simulink model "DPGandLQRIdentHandK"  (R2025b)
settings: Solver=VariableStepAuto  StartTime=0.0  StopTime=60000  FixedStep=1e-3  MaxStep=1e-3  RelTol=1e-3
values from neighbouring files (symbols this model uses):
  A = [1.0000    0.0099 ... (first row only)    [DPGandLQRIdentHandK.m]    (also in DPGandLQR_usingDlfevel.m = [1.0000, 0.0099; DPGandLQRsimOnlyIdentH.m)
  B = [4.9503e-05 ... (first row only)    [DPGandLQRIdentHandK.m]    (also in DPGandLQR_usingDlfevel.m; DPGandLQRsimOnlyIdentH.m)
  C = eye(size(A))    [DPGandLQRIdentHandK.m]    (also in DPGandLQRsimOnlyIdentH.m)
  H_critic = (H_critic + H_critic') / 2    [DPGandLQRIdentHandK.m]    (also in DPGandLQR_usingDlfevel.m = 0.5 * (H_critic + H_critic'); DPGandLQRsimOnlyIdentH.m)
  Herror = [1 1 1;1  1 1;1 1 1]*20    [DPGandLQRIdentHandK.m]    (also in DPGandLQRsimOnlyIdentH.m)
  Q = eye(2)    [DPGandLQRIdentHandK.m]    (also in DPGandLQR_usingDlfevel.m; DPGandLQRsimOnlyIdentH.m)
  R = 1    [DPGandLQRIdentHandK.m]    (also in DPGandLQR_usingDlfevel.m; DPGandLQRsimOnlyIdentH.m)
undefined symbols (not defined in the file or in its folder): K_lqr, magnitude, P_star
libraries: simulink x2
settings Model: PacingRate=1000  Creator=17547  LastModifiedBy=17547

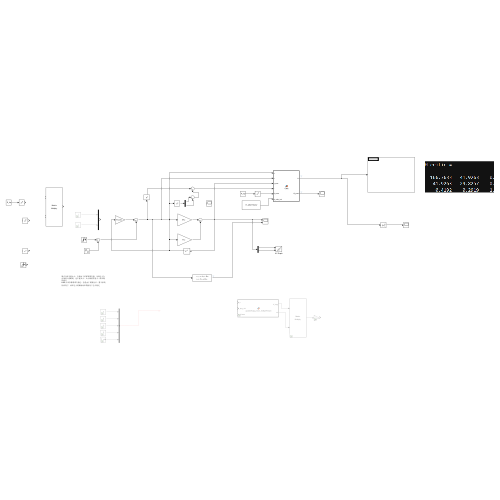
[thumbnail: Simulink's stored preview of the top-level diagram]
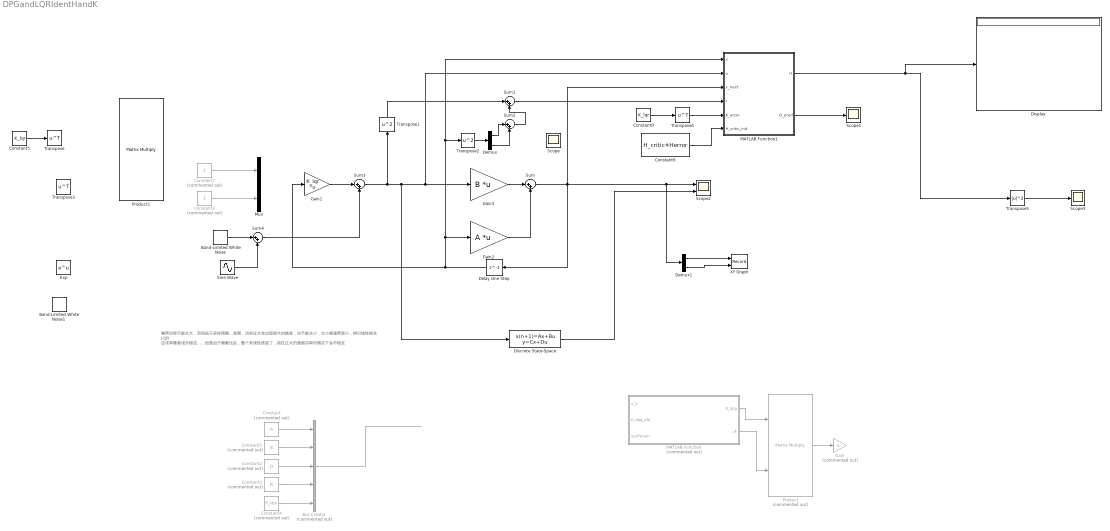
== system DPGandLQRIdentHandK ==
  note: 噪声功率不能太大，否则由于采样周期有限，功率过大会出现很大的跳变；也不能太小，太小频谱带宽小，辨识线性相关
      | LQR 应该李雅普诺夫稳定，但是由于离散化后，整个系统性质变了，故在过大的激励功率的情况下会不稳定
  Band-Limited White Noise : simulink/Sources/Band-Limited White Noise  Cov=[0.004]  Ts=0.01  seed=[23341]
  Band-Limited White Noise1 : simulink/Sources/Band-Limited White Noise  Cov=[0.1]  Ts=0.01  seed=[23341]
  Bus Creator : BusCreator  Commented=on  Inputs=5  OutDataTypeStr=Bus: sysParamType
  Constant : Constant  Commented=on  Value=A
  Constant1 : Constant  Commented=on  Value=B
  Constant2 : Constant  Commented=on  Value=Q
  Constant3 : Constant  Commented=on  Value=R
  Constant4 : Constant  Commented=on  Value=P_star
  Constant5 : Constant  Value=K_lqr
  Constant6 : Constant  Value=H_critic+Herror
  Constant7 : Constant  Commented=on
  Constant8 : Constant  Commented=on
  Constant9 : Constant  Value=K_lqr
  Delay One Step : Delay  DelayLength=1
  Demux : Demux  Outputs=2
  Demux1 : Demux  Outputs=2
  Discrete State-Space : DiscreteStateSpace  A=A  B=B  C=C  D=zeros(size(B))  SampleTime=-1
  Display : Display
  Exp : Math
  Gain : Gain  Commented=on  Gain=-1
  Gain1 : Gain  Gain=K_lqr  Multiplication=Matrix(K*u) (u vector)
  Gain2 : Gain  Gain=A  Multiplication=Matrix(K*u)
  Gain3 : Gain  Gain=B  Multiplication=Matrix(K*u)
  MATLAB Function : MATLAB Function  Commented=on  TreatAsAtomicUnit=on
  MATLAB Function1 : MATLAB Function  TreatAsAtomicUnit=on
  Mux : Mux  Inputs=2
  Product : Product  Commented=on  Multiplication=Matrix(*)
  Product1 : Product  Multiplication=Matrix(*)
  Scope : Scope
      settings: ActiveDisplayYMinimum=-1  ActiveDisplayYMaximum=1
  Scope1 : Scope
      settings: ActiveDisplayYMinimum=-2.5586551509886442  ActiveDisplayYMaximum=55.587001955566855  DataLoggingVariableName=ScopeData2
  Scope2 : Scope  NumInputPorts=2
      settings: ActiveDisplayYMinimum=-0.91908359035727893  ActiveDisplayYMaximum=0.94235805810106676
  Scope3 : Scope
      settings: ActiveDisplayYMinimum=-3486.71302595445  ActiveDisplayYMaximum=31381.269885559039  DataLoggingVariableName=ScopeData3
  Sine Wave : Sin  Amplitude=2  Frequency=2  SampleTime=0
  Sum{,1..4} (5 alike) : Sum  Inputs=|++
  Transpose : Math  Operator=transpose
  Transpose1 : Math  Operator=square
  Transpose2 : Math  Operator=square
  Transpose3 : Math  Operator=transpose
  Transpose4 : Math  Operator=transpose
  Transpose5 : Math  Operator=magnitude^2
  XY Graph : Record  NumPorts=2.0  FileSettingsInternal="{\"entries\":[{\"content\":{\"excelSettings\":{\"content\":{},\"type\":\"Streamout.ExcelSettings\"},\"parquetSettings\":{\"content\":{},\"type\":\"Streamout.ParquetSettings\"}},\"type\":\"Streamout.FileSettingStorage\",\"uuid\":\"\"}],\"packageUris\":[\"http:\\/\\/schema.mathworks.com\\/mf0\\/streamout_blocks\\/R2020a\"],\"version\":\"1.0\"}"  FrameSettings=[0, 0]  Layout=[1 1]  SignalsInternal="{\"entries\":[{\"content\":{\"signals\":[{\"content\":{\"blockPath\":[],\"dimensions\":[1],\"domain\":\"\",\"lineColor\":\"#a2142f\",\"plots\":[ 1 ],\"port\":1,\"signalID\":1,\"signalName\":\"XY Graph:1\"},\"type\":\"RecordBlkView.Signal\",\"uuid\":\"\"},{\"content\":{\"blockPath\":[],\"dimensions\":[1],\"domain\":\"\",\"lineColor\":\"#139fff\",\"plots\":[ 1 ],\"port\":2,\"signalID\":2,\"signalName\":\"XY Graph:2\"},\"type\":\"RecordBlkView.Signal\",\"uuid\":\"\"}]},\"type\":\"RecordBlkView.InputSignals\",\"uuid\":\"\"}],\"packageUris\":[\"http:\\/\\/schema.mathworks.com\\/mf0\\/streamout_blocks\\/R2020a\"],\"version\":\"1.0\"}"  VisualizationBindings="{\"xyplotplugin\":{\"info\":[{\"series\":[{\"bindingParametersList\":[{\"parameter\":\"X-Axis\",\"signalID\":1,\"signalName\":\"XY Graph:1\"},{\"parameter\":\"Y-Axis\",\"signalID\":2,\"signalName\":\"XY Graph:2\"}],\"seriesID\":0}],\"subplotID\":1}]}}"  CompatibilityTag=XY
  wires:
  Constant2/1 -> Bus Creator/3
  Constant1/1 -> Bus Creator/2
  Constant4/1 -> Bus Creator/5
  Bus Creator/1 -> ?
  Constant/1 -> Bus Creator/1
  Constant3/1 -> Bus Creator/4
  MATLAB Function/2(uk) -> Product/2
  Product/1 -> Gain/1
  MATLAB Function/1(K_dpg) -> Product/1
  Constant5/1 -> Transpose/1
  Constant6/1 -> MATLAB Function1/6(H_critic_init)
  Gain3/1 -> Sum/1
  Gain2/1 -> Sum/2
  Delay One Step/1 -> Gain2/1, Transpose2/1, MATLAB Function1/1(x), Gain1/1
  Sum/1 -> MATLAB Function1/3(x_next), Demux1/1, Scope2/1, Delay One Step/1
  Sum3/1 -> Discrete State-Space/1, Gain3/1, MATLAB Function1/2(u), Transpose1/1
  Sum1/1 -> MATLAB Function1/4(r)
  Transpose1/1 -> Sum1/1
  Transpose2/1 -> Demux/1
  Constant9/1 -> Transpose4/1
  Demux/2 -> Sum2/2
  Demux/1 -> Sum2/1
  Sum2/1 -> Sum1/2
  Constant8/1 -> Mux/2
  Constant7/1 -> Mux/1
  Transpose4/1 -> MATLAB Function1/5(K_actor)
  Discrete State-Space/1 -> Scope2/2
  Gain1/1 -> Sum3/1
  MATLAB Function1/2(Q_pred) -> Scope1/1
  MATLAB Function1/1(H) -> Transpose5/1, Display/1
  Transpose5/1 -> Scope3/1
  Band-Limited White Noise/1 -> Sum4/1
  Sum4/1 -> Sum3/2
  Sine Wave/1 -> Sum4/2
  Demux1/2 -> XY Graph/2
  Demux1/1 -> XY Graph/1

== matlab function DPGandLQRIdentHandK/MATLAB Function1 ==
  data: x input; u input; x_next input; r input; K_actor input; H output; H_critic_init input; Q_pred output
function [H,Q_pred] = Critic(x, u, x_next, r, K_actor, H_critic_init)
 
    persistent H_critic  % 生命周期持续到仿真结束
    if isempty(H_critic)
        H_critic = H_critic_init;  % 用输入端口设置初值
    end

    gamma = 1;
    alpha_critic = 0.005;
    % 更新 Critic (Policy Evaluation, TD-Learning) ---
    
    z = [x; u];
    
    % 目标策略 (Target Policy): 评估当前 Actor 的纯策略 (无噪声)
    u_next = -K_actor * x_next; 
    z_next = [x_next; u_next];
    
    % 计算 TD 误差: 预测值 vs 目标值 (半梯度法，不对目标求导)
    Q_pred = z' * H_critic * z;
    Q_target = r + gamma * (z_next' * H_critic * z_next);
    delta = Q_pred - Q_target;
    
    %  Critic 梯度: \nabla_H Loss = delta * z * z'    % deepseek J = v'Hv  对H求梯度  等于什么
    TDerrwithG = delta * (z * z');

    % 梯度下降更新 H，并强制对称化
    H_critic = H_critic - alpha_critic * (TDerrwithG);
    H_critic = (H_critic + H_critic') / 2; 
    H = H_critic;
end

== matlab function DPGandLQRIdentHandK/MATLAB Function ==
  data: x_k input; K_dpg output; K_dpg_old input; sysParam input Bus: sysParamType; uk output
function [K_dpg,uk] = updateKdpg_from_fullSysParam(x_k,K_dpg_old,sysParam)
    A = sysParam.A;
    B = sysParam.B;
    Q = sysParam.Q;
    R = sysParam.R;
    P_star = sysParam.P_star;  % lqr直接给出。
    learning_rate = 0.01;

    u_k = -K_dpg_old * x_k;
    % 1. 计算 Q* 对 u 的梯度: \nabla_u Q^*(x_k, u)
    % 公式: 2*R*u + 2*B'*P*(A*x_k + B*u)
    grad_u_Q = 2 * R * u_k + 2 * B' * P_star * (A * x_k + B * u_k);
    
    % 2. 计算链式法则得到的策略梯度对 K 的偏导: \nabla_K J(K)
    % 因为我们要最小化代价值 (Minimize Cost)，所以直接使用你的推导公式：
    % \nabla_K C_sample = - \nabla_u Q^* * x_k'
    grad_K_sample = -grad_u_Q * x_k'; 
   
    
    % 梯度下降更新 K (目标是最小化 Cost)
    K_dpg = K_dpg_old - learning_rate * grad_K_sample;
end
